simulink model "TP1_SIM_R3FMO_ctrl"  (R2023b)
settings: Solver=ode23s  StartTime=0.0  StopTime=0.2  RelTol=1e-3  EnableMultiTasking=on
values from neighbouring files (symbols this model uses):
  deltat = deltat_2    (= 35)    [tp1_a.m]    (also in workspace.mat = 5)
  theta = 3    [tp1_a.m]    (also in workspace.mat = 1)
libraries: spsVoltageMeasurementLib x4, spsThyristorLib x3, spsMeanLib x2, spsBreakerLib x1, spsCurrentMeasurementLib x1, spsGroundLib x1, spsSeriesRLCLoadLib x1, spsThreePhaseProgrammableVoltageSourceLib x1, spspowerguiLib x1
settings Model: Creator=Moni  LastModifiedBy=Amadeo
settings SolverCC: AlgebraicLoopSolver=TrustRegion
settings DataIOCC: SaveFormat=Array  SaveState=on  ReturnWorkspaceOutputs=off
settings OptimizationCC: LifeSpan=inf
settings DebuggingCC: SolverPrmCheckMsg=warning  UnconnectedInputMsg=warning  UnconnectedOutputMsg=warning  UnconnectedLineMsg=warning  SFUnexpectedBacktrackingDiag=warning  SFNoUnconditionalDefaultTransitionDiag=warning  SFExecutionAtInitializationDiag=none  ArithmeticOperatorsInVariantConditions=warning
settings HardwareCC: ProdBitPerPointer=32  ProdBitPerSizeT=32  ProdBitPerPtrDiffT=32  ProdLargestAtomicFloat=None  ProdIntDivRoundTo=Undefined  ProdEndianess=Unspecified  ProdWordSize=32  ProdHWDeviceType=32-bit Generic
settings ModelReferenceCC: EnableRefExpFcnMdlSchedulingChecks=on  PropagateSignalLabelsOutOfModel=off
settings SFSimCC: SimUseLocalCustomCode=off  CustomCodeUndefinedFunction=UseInterfaceOnly
settings RTWCC: RTWUseLocalCustomCode=off
settings CodeAppCC: StateflowObjectComments=on
settings GRTTargetCC: TargetLangStandard=C89/C90 (ANSI)
settings ConfigComp: CovMetricSettings=dw  CovSaveCumulativeToWorkspaceVar=on  CovSaveSingleToWorkspaceVar=on  CovExternalEMLEnable=off  CovSFcnEnable=off
settings SimscapeCC: SimscapeNormalizeSystem=off

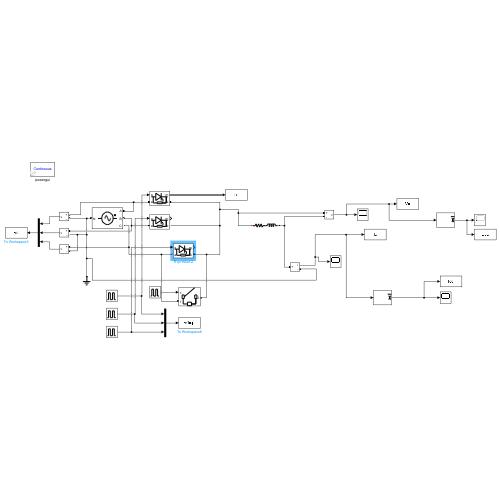
[thumbnail: Simulink's stored preview of the top-level diagram]
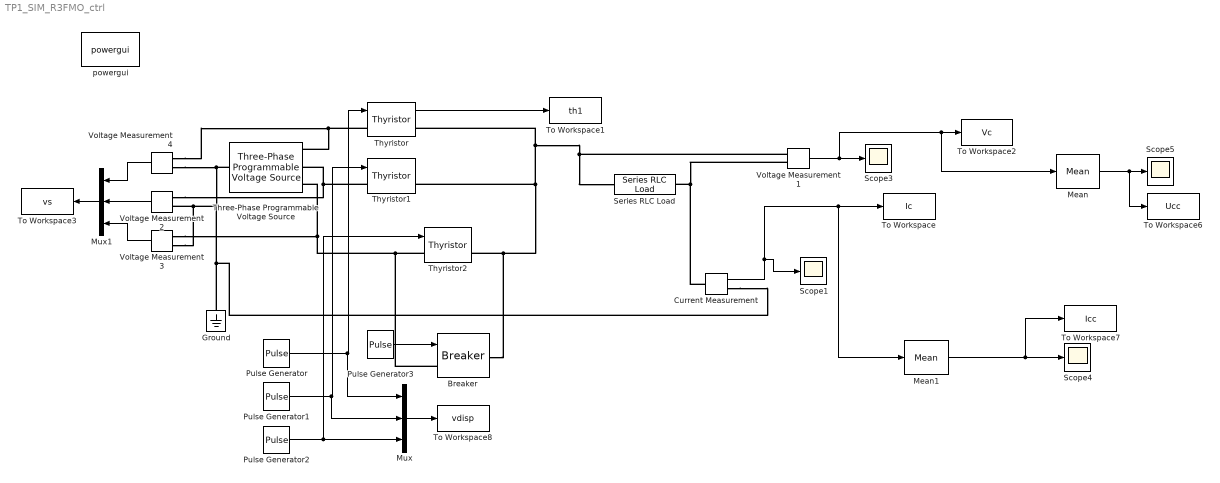
== system TP1_SIM_R3FMO_ctrl ==
  Breaker : spsBreakerLib/Breaker  InitialState=0  SwitchingTimes="[1/60  5/60]"  External=on  BreakerResistance=0.01  SnubberResistance=1e6  SnubberCapacitance=inf  Measurements=None  MoreParameters=on  NoBreakLoop=off
  Current Measurement : spsCurrentMeasurementLib/Current Measurement  PhasorSimulation=off  OutputType=Complex  PSBequivalent=0
  Ground : spsGroundLib/Ground  LConnTagsString=a
  Mean : spsMeanLib/Mean  Freq=50  Vinit=0  Ts=0
  Mean1 : spsMeanLib/Mean  Freq=50  Vinit=0  Ts=0
  Mux : Mux  Inputs=3
  Mux1 : Mux  Inputs=3
  Pulse Generator : DiscretePulseGenerator  PulseType=Time based  Period=.02  PulseWidth=deltat  PhaseDelay=t(theta,1)
  Pulse Generator1 : DiscretePulseGenerator  PulseType=Time based  Period=.02  PulseWidth=deltat  PhaseDelay=t(theta,2)
  Pulse Generator2 : DiscretePulseGenerator  PulseType=Time based  Period=.02  PulseWidth=deltat  PhaseDelay=t(theta,3)
  Pulse Generator3 : DiscretePulseGenerator  PulseType=Time based  Period=10  PulseWidth=50  PhaseDelay=.5
  Scope{1,3..5} (4 alike) : Scope
  Series RLC Load : spsSeriesRLCLoadLib/Series RLC Load  LConnTagsString=a  RConnTagsString=__new0  NominalVoltage=220  NominalFrequency=50  ActivePower=P  InductivePower=Q  CapacitivePower=0  Setx0=off  InitialVoltage=0  SetiL0=off  InitialCurrent=0  Measurements=None  LoadType=constant Z
  Three-Phase Programmable Voltage Source : spsThreePhaseProgrammableVoltageSourceLib/Three-Phase Programmable Voltage Source  PositiveSequence="[380  0 50]"  VariationEntity=None  VariationType=Table of time-amplitude pairs  VariationTypeAlt=Step  VariationStep=0.5  VariationRate=10  VariationMagnitude=0.3  VariationFrequency=2  VariationTiming=[1 2]  VariationPhaseA=off  Amplitudes=[1 0.8 1.2 1.0]  TimeValues=[0 0.1 0.15 0.2]  HarmonicGeneration=off  HarmonicA=[3 0.2 -25 0]  HarmonicB=[2 0.15 35 2]  Timing="[0.05  3]"  BusType=swing  Pref=0  Qref=0  Qmin=-inf  Qmax=inf
  Thyristor : spsThyristorLib/Thyristor  Ron=0.001  Lon=0  Vf=0.8  IC=0  Rs=400  Cs=C_snubber  Measurements=on
  Thyristor1 : spsThyristorLib/Thyristor  Ron=0.001  Lon=0  Vf=0.8  IC=0  Rs=400  Cs=C_snubber  Measurements=on
  Thyristor2 : spsThyristorLib/Thyristor  Ron=0.001  Lon=0  Vf=0.8  IC=0  Rs=400  Cs=C_snubber  Measurements=on
  To Workspace : ToWorkspace  VariableName=Ic  SampleTime=-1
  To Workspace1 : ToWorkspace  VariableName=th1  SampleTime=-1
  To Workspace2 : ToWorkspace  VariableName=Vc  SampleTime=-1
  To Workspace3 : ToWorkspace  VariableName=vs  SampleTime=-1
  To Workspace6 : ToWorkspace  VariableName=Ucc  SampleTime=-1
  To Workspace7 : ToWorkspace  VariableName=Icc  SampleTime=-1
  To Workspace8 : ToWorkspace  VariableName=vdisp  SampleTime=-1
  Voltage Measurement{1..4} (4 alike) : spsVoltageMeasurementLib/Voltage Measurement  PhasorSimulation=off  OutputType=Complex  PSBequivalent=0
  powergui : spspowerguiLib/powergui  Priority=1  SimulationMode=Continuous  SampleTime=50e-6  frequency=60  Iterations=50  frequencyindice=50  Pbase=100e6  ErrMax=1e-4  UnitsV=kV  UnitsW=MW  buscounter=0  FunctionMessages=off  echomessages=off  EnableUseOfTLC=off  CurrentSourceSwitches=on  DisableSnubberDevices=off  DisableRonSwitches=off  DisableVfSwitches=off  DisplayEquations=off  AutomaticDiscreteSolvers=off  SolverType=Tustin  Interpol=off  ExternalGateDelay=off  methode=off  Ts=0  x0status=blocks  SPID=off  SwTol=0  HookPort=off  NonlinearTolerance=1e-4  nMaxIteration=100  ContinueOnMaxIteration=off  RestoreLinks=warning  ResistiveCurrentMeasurement=off  Frange=[0:2:500]  Ylog=off  Xlog=on  ShowGrid=off  save=off  variable=ZData  structure=Vc  ZoomFFT=off  StartTime=0.3  cycles=3  DisplayStyle=1  fundamental=50  FreqAxis=off  MaxFrequency=500  frequencyindicesteady=1  RmsSteady=1  display=off
  wires:
  Current Measurement/1 -> Scope1/1, Mean1/1, To Workspace/1
  Thyristor/1 -> To Workspace1/1
  Voltage Measurement1/1 -> Mean/1, To Workspace2/1, Scope3/1
  Pulse Generator/1 -> Mux/1, Thyristor/1
  Pulse Generator1/1 -> Mux/2, Thyristor1/1
  Pulse Generator2/1 -> Thyristor2/1, Mux/3
  Mean1/1 -> To Workspace7/1, Scope4/1
  Mean/1 -> To Workspace6/1, Scope5/1
  Pulse Generator3/1 -> Breaker/1
  Voltage Measurement2/1 -> Mux1/2
  Voltage Measurement3/1 -> Mux1/3
  Mux/1 -> To Workspace8/1
  Voltage Measurement4/1 -> Mux1/1
  Mux1/1 -> To Workspace3/1
  connections:
  Thyristor/LConn1 -- Three-Phase Programmable Voltage Source/RConn1 -- Voltage Measurement4/LConn1
  Thyristor1/LConn1 -- Voltage Measurement2/LConn1 -- Three-Phase Programmable Voltage Source/RConn2
  Thyristor2/LConn1 -- Breaker/LConn1 -- Three-Phase Programmable Voltage Source/RConn3 -- Voltage Measurement3/LConn1
  Breaker/RConn1 -- Thyristor2/RConn1 -- Thyristor1/RConn1 -- Thyristor/RConn1 -- Voltage Measurement1/LConn1 -- Series RLC Load/LConn1
  Current Measurement/LConn1 -- Voltage Measurement1/LConn2 -- Series RLC Load/RConn1
  Ground/LConn1 -- Current Measurement/RConn1 -- Voltage Measurement4/LConn2 -- Three-Phase Programmable Voltage Source/LConn1 -- Voltage Measurement3/LConn2 -- Voltage Measurement2/LConn2
